simulink model "DDCurrentController"  (R2020a)
settings: Solver=FixedStepAuto  StartTime=0.0  StopTime=10.0  RelTol=1e-3
settings Model: DataDictionary=PCS_Simulation_EnviromentDD.sldd  Creator=ykamatan  LastModifiedBy=ykamatan
settings OptimizationCC: DefaultParameterBehavior=Inlined  EnhancedBackFolding=on  PassReuseOutputArgsAs=Individual arguments  ZeroExternalMemoryAtStartup=off  ZeroInternalMemoryAtStartup=off  OptimizeBlockOrder=speed  DifferentSizesBufferReuse=on  OptimizationCustomize=off  EfficientTunableParamExpr=on
settings DebuggingCC: ParameterTunabilityLossMsg=error
settings ModelReferenceCC: ModelReferenceNumInstancesAllowed=Single
settings SFSimCC: MATLABDynamicMemAlloc=off
settings RTWCC: SystemTargetFile=ert.tlc  TemplateMakefile=ert_default_tmf
settings CodeAppCC: ForceParamTrailComments=on  IgnoreCustomStorageClasses=off  OperatorAnnotations=on  SimulinkDataObjDesc=on  SFDataObjDesc=on  InsertBlockDesc=on
settings ERTTargetCC: TargetLangStandard=C99 (ISO)  GenerateSampleERTMain=on  InlinedParameterPlacement=NonHierarchical  ERTCustomFileTemplate=example_file_process.tlc

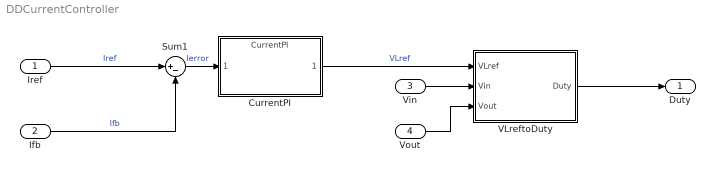
== system DDCurrentController ==
  Iref : Inport
  Ifb : Inport  Port=2
  Vin : Inport  Port=3
  Vout : Inport  Port=4
  CurrentPI : ModelReference  ModelNameDialog=CurrentPI  SimulationMode=Normal  ModelReferenceVersion=1.24
  Sum1 : Sum  Inputs=|+-
  VLreftoDuty : Subsystem  TreatAsAtomicUnit=on
  Duty : Outport
  wires:
  Sum1/1 -> CurrentPI/1  "Ierror"
  Ifb/1 -> Sum1/2  "Ifb"
  Iref/1 -> Sum1/1  "Iref"
  CurrentPI/1 -> VLreftoDuty/1(VLref)  "VLref"
  Vin/1 -> VLreftoDuty/2(Vin)
  Vout/1 -> VLreftoDuty/3(Vout)
  VLreftoDuty/1(Duty) -> Duty/1

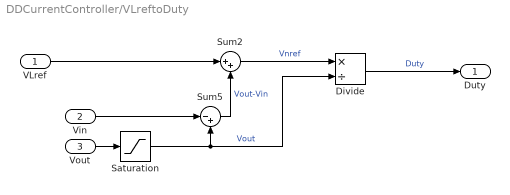
== system DDCurrentController/VLreftoDuty ==
  VLref : Inport
  Vin : Inport  Port=2
  Vout : Inport  Port=3
  Divide : Product  Inputs=*/
  Saturation : Saturate  UpperLimit=inf  LowerLimit=1
  Sum2 : Sum  Inputs=|++
  Sum5 : Sum  Inputs=|-+
  Duty : Outport
  wires:
  Vin/1 -> Sum5/1
  Sum2/1 -> Divide/1  "Vnref"
  Saturation/1 -> Divide/2, Sum5/2  "Vout"
  Sum5/1 -> Sum2/2  "Vout-Vin"
  Vout/1 -> Saturation/1
  VLref/1 -> Sum2/1
  Divide/1 -> Duty/1  "Duty"
